simulink model "model_1d"  (R2019b)
settings: Solver=VariableStepAuto  StartTime=0.0  StopTime=simulation_time  RelTol=1e-3
values from neighbouring files (symbols this model uses):
  duty_cycle = 0.5    [params.m]
  Gs = tf(K, [tau 1])    [params.m]
  T0 = 27    [params.m]
settings Model: Creator=adityaaaap  LastModifiedBy=adityaaaap

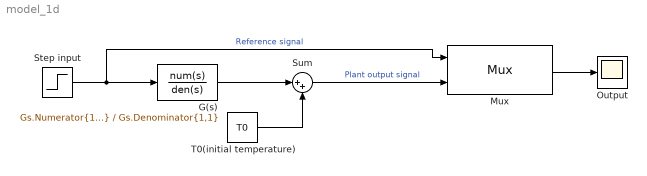
== system model_1d ==
  " T0(initial temperature)" : Constant  Value=T0
  G(s) : TransferFcn  Numerator=Gs.Numerator{1,1}  Denominator=Gs.Denominator{1,1}
  Mux : Mux  Inputs=2
      settings: DisplayOption=signals
  Output : Scope
  Step input : Step  Time=0  After=1*duty_cycle  SampleTime=0.1
  Sum : Sum  Inputs=|++
  wires:
  Step input/1 -> Mux/1, G(s)/1  "Reference signal"
  G(s)/1 -> Sum/1
  " T0(initial temperature)"/1 -> Sum/2
  Sum/1 -> Mux/2  "Plant output signal"
  Mux/1 -> Output/1
